simulink model "speedControlSimulation"  (R2024b)
settings: Solver=FixedStepAuto  StartTime=0.0  StopTime=Tend  FixedStep=Tsim  RelTol=1e-4
values from neighbouring files (symbols this model uses):
  b = 4.28e-6    (= 4.28e-06)    [setup.m]    (also in test.m)
  J_z = 29.54e-6    (= 2.954e-05)    [setup.m]
  Ki_speed = omega_b_speed*b    (= 0.00268920331147)    [setup.m]
  Kp_speed = omega_b_speed*J_z    (= 0.0185605293974)    [setup.m]
  speed_cmd = 3000    [setup.m]
  Ts = 1e-4    (= 0.0001)    [setup.m]    (also in test.m = 0.001)
undefined symbols (not defined in the file or in its folder): DiscIntNeverNeededParam
settings Model: Creator=puroh  LastModifiedBy=tnoguchi
settings OptimizationCC: DefaultParameterBehavior=Inlined  EnhancedBackFolding=on  PassReuseOutputArgsAs=Individual arguments  ZeroExternalMemoryAtStartup=off  ZeroInternalMemoryAtStartup=off  OptimizeBlockOrder=speed  DifferentSizesBufferReuse=on  EfficientTunableParamExpr=on
settings DebuggingCC: ParameterTunabilityLossMsg=error  UnconnectedInputMsg=warning  UnconnectedOutputMsg=warning  UnconnectedLineMsg=warning
settings ModelReferenceCC: EnableRefExpFcnMdlSchedulingChecks=on
settings SFSimCC: MATLABDynamicMemAlloc=off
settings RTWCC: Description=Embedded Coder  SystemTargetFile=ert.tlc  TemplateMakefile=ert_default_tmf  GPUComputeCapability=3.5  DLArmComputeVersion=19.05
settings CodeAppCC: ForceParamTrailComments=on  IgnoreCustomStorageClasses=off  OperatorAnnotations=on  SimulinkDataObjDesc=on  SFDataObjDesc=on  InsertBlockDesc=on
settings ERTTargetCC: TargetLangStandard=C99 (ISO)  ERTCustomFileTemplate=example_file_process.tlc  DynamicArrayContainerType=coder::array
settings ConfigComp: CovBoundaryAbsTol=1.0e-5

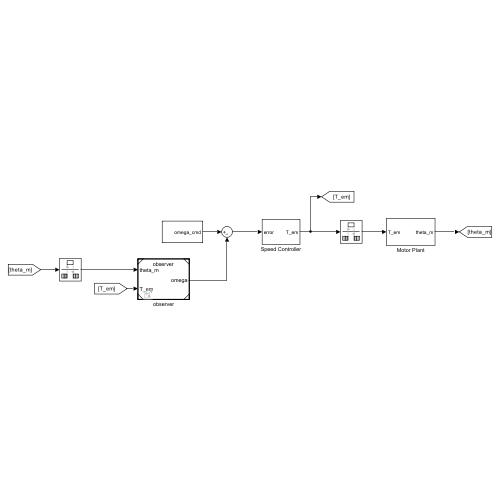
[thumbnail: Simulink's stored preview of the top-level diagram]
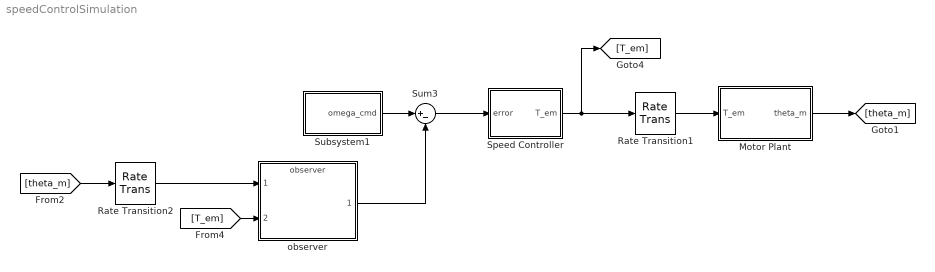
== system speedControlSimulation ==
  Motor Plant : Subsystem
  Rate Transition1 : RateTransition
  Rate Transition2 : RateTransition  OutPortSampleTime=Ts
  Speed Controller : Subsystem
  Subsystem1 : Subsystem
  Sum3 : Sum  Inputs=|+-
  observer : ModelReference  ModelNameDialog=observer  SimulationMode=Normal  ModelReferenceVersion=10.14
  wires:
  [theta_m] -> Rate Transition2/1
  Rate Transition1/1 -> Motor Plant/1(T_em)
  Motor Plant/1(theta_m) -> [theta_m]
  Speed Controller/1(T_em) -> Rate Transition1/1, [T_em]
  Subsystem1/1(omega_cmd) -> Sum3/1
  Sum3/1 -> Speed Controller/1(error)
  Rate Transition2/1 -> observer/1
  observer/1 -> Sum3/2
  [T_em] -> observer/2

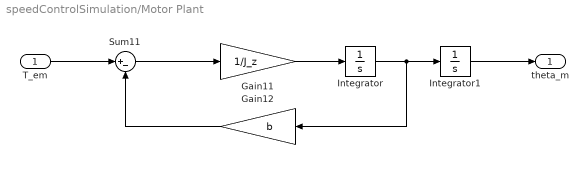
== system speedControlSimulation/Motor Plant ==
  T_em : Inport
  Gain11 : Gain  Gain=1/J_z
  Gain12 : Gain  Gain=b
  Integrator : Integrator
  Integrator1 : Integrator  WrapState=on  WrappedStateUpperValue=2*pi  WrappedStateLowerValue=0
  Sum11 : Sum  Inputs=|+-
  theta_m : Outport
  wires:
  Integrator1/1 -> theta_m/1
  Gain12/1 -> Sum11/2
  Integrator/1 -> Gain12/1, Integrator1/1
  T_em/1 -> Sum11/1
  Gain11/1 -> Integrator/1
  Sum11/1 -> Gain11/1

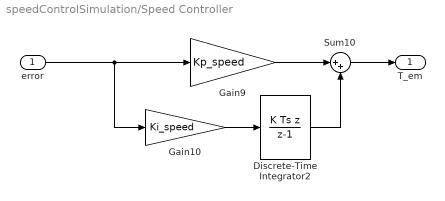
== system speedControlSimulation/Speed Controller ==
  error : Inport
  Discrete-Time Integrator2 : DiscreteIntegrator  IntegratorMethod=Integration: Backward Euler  SampleTime=-1  ICPrevOutput=DiscIntNeverNeededParam  ICPrevScaledInput=DiscIntNeverNeededParam
  Gain10 : Gain  Gain=Ki_speed
  Gain9 : Gain  Gain=Kp_speed
  Sum10 : Sum  Inputs=|++
  T_em : Outport
  wires:
  Discrete-Time Integrator2/1 -> Sum10/2
  Gain9/1 -> Sum10/1
  Gain10/1 -> Discrete-Time Integrator2/1
  error/1 -> Gain10/1, Gain9/1
  Sum10/1 -> T_em/1

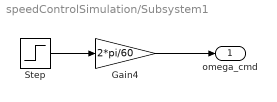
== system speedControlSimulation/Subsystem1 ==
  Gain4 : Gain  Gain=2*pi/60
  Step : Step  Time=0.04  After=speed_cmd  SampleTime=Ts
  omega_cmd : Outport
  wires:
  Step/1 -> Gain4/1
  Gain4/1 -> omega_cmd/1
